simulink model "ResourceAllocation"  (R2026a)
settings: Solver=VariableStepAuto  StopTime=20.0

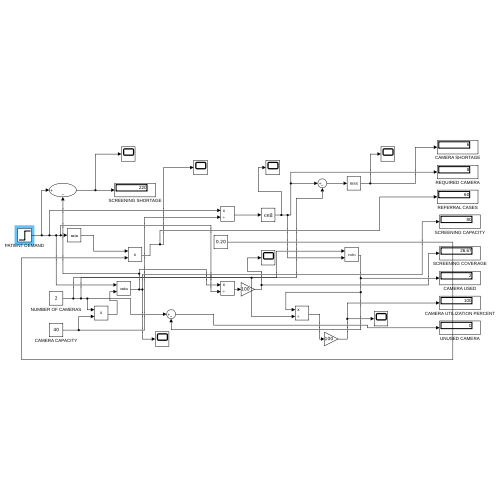
[thumbnail: Simulink's stored preview of the top-level diagram]
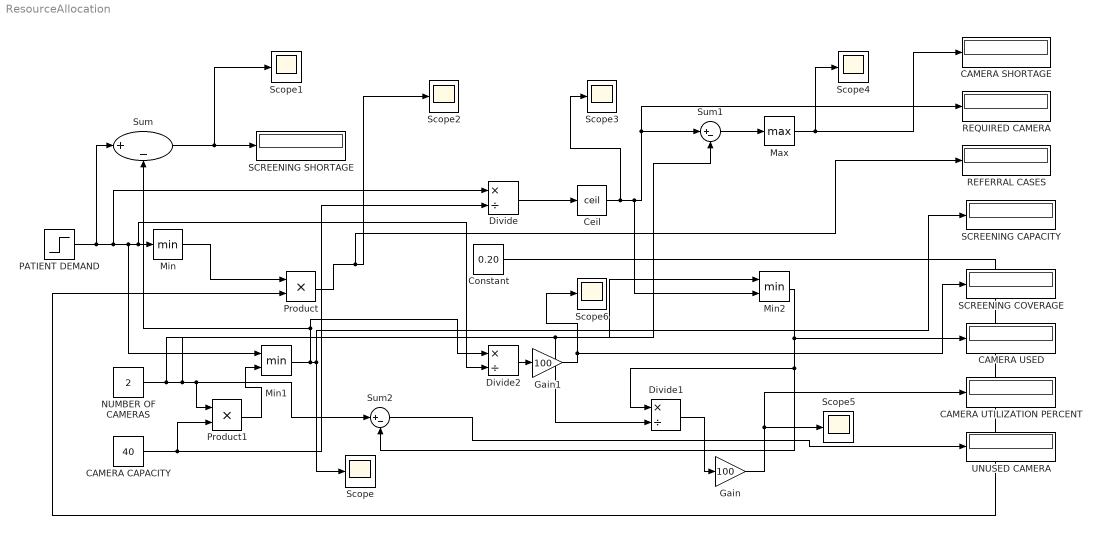
== system ResourceAllocation ==
  CAMERA CAPACITY : Constant  Value=40
  CAMERA SHORTAGE : Display
  CAMERA USED : Display
  CAMERA UTILIZATION PERCENT : Display
  Ceil : Rounding  Operator=ceil
  Constant : Constant  Value=0.20
  Divide : Product  Inputs=*/
  Divide1 : Product  Inputs=*/
  Divide2 : Product  Inputs=*/
  Gain : Gain  Gain=100
  Gain1 : Gain  Gain=100
  Max : MinMax  Function=max
  Min : MinMax
  Min1 : MinMax  Inputs=2
  Min2 : MinMax  Inputs=2
  NUMBER OF CAMERAS : Constant  Value=2
  PATIENT DEMAND : Step  Time=10  InitialValue=100  FinalValue=300  SampleTime=0
  Product : Product
  Product1 : Product
  REFERRAL CASES : Display
  REQUIRED CAMERA : Display
  SCREENING CAPACITY : Display
  SCREENING COVERAGE : Display
  SCREENING SHORTAGE : Display
  Scope{,1..6} (7 alike) : Scope
      Scope settings: ActiveDisplayYMinimum=14.40910628577182  ActiveDisplayYMaximum=93.569197762172081
      Scope1 settings: ActiveDisplayYMinimum=-81.081561233003612  ActiveDisplayYMaximum=104.73009369483711
      Scope2 settings: ActiveDisplayYMinimum=-15.977162673711206  ActiveDisplayYMaximum=38.391692541208059  DataLoggingVariableName=ScopeData2
      Scope3 settings: ActiveDisplayYMinimum=1.75  ActiveDisplayYMaximum=4.25  DataLoggingVariableName=ScopeData3
      Scope4 settings: ActiveDisplayYMinimum=-0.24999999999999994  ActiveDisplayYMaximum=2.25  DataLoggingVariableName=ScopeData4
      Scope5 settings: ActiveDisplayYMinimum=90  ActiveDisplayYMaximum=110  DataLoggingVariableName=ScopeData5
      Scope6 settings: ActiveDisplayYMinimum=47.5  ActiveDisplayYMaximum=105.83333333333333  DataLoggingVariableName=ScopeData6
  Sum : Sum  Inputs=|+-
  Sum1 : Sum  Inputs=|+-
  Sum2 : Sum  Inputs=|+-
  UNUSED CAMERA : Display
  wires:
  Min/1 -> Product/1
  Constant/1 -> Product/2
  Product/1 -> Scope2/1, REFERRAL CASES/1
  PATIENT DEMAND/1 -> Divide2/2, Min/1, Min1/1, Divide/1, Sum/1
  Sum/1 -> Scope1/1, SCREENING SHORTAGE/1
  NUMBER OF CAMERAS/1 -> Divide1/2, Sum1/2, Sum2/1, Product1/1, Min2/1
  CAMERA CAPACITY/1 -> Divide/2, Product1/2
  Product1/1 -> Min1/2
  Min1/1 -> Sum/2, Divide2/1, Scope/1, SCREENING CAPACITY/1
  Divide/1 -> Ceil/1
  Ceil/1 -> Scope3/1, Min2/2, Sum1/1, REQUIRED CAMERA/1
  Sum1/1 -> Max/1
  Min2/1 -> Divide1/1, Sum2/2, CAMERA USED/1
  Sum2/1 -> UNUSED CAMERA/1
  Divide1/1 -> Gain/1
  Gain/1 -> Scope5/1, CAMERA UTILIZATION PERCENT/1
  Divide2/1 -> Gain1/1
  Gain1/1 -> Scope6/1, SCREENING COVERAGE/1
  Max/1 -> Scope4/1, CAMERA SHORTAGE/1
